simulink model "Wind_Turbine_Model"  (R2023a)
settings: Solver=VariableStepAuto  StartTime=0.0  StopTime=65  RelTol=1e-3
values from neighbouring files (symbols this model uses):
  Cbus = 80e-3*n_wt_agg*u^2    (= 1.33333333333)    [param.m]
  D = 1e-3    (= 0.001)    [param.m]
  f = 50    [param.m]
  Fs = Vs * sqrt(2/3)/(2*pi*f)    [param.m]
  fsw = 4e3    (= 4000)    [param.m]
  Idr_rated = sqrt(2)*Is    [param.m]
  J = 127*n_wt_agg    (= 19050)    [param.m]
  ki_id = (wni^2)*Lr*sigma    (= 3.27733001332)    [param.m]
  ki_idg = (wnig^2)*Lg    (= 0.263189450696)    [param.m]
  ki_iq = ki_id    (= 3.27733001332)    [param.m]
  ki_iqg = ki_idg    (= 0.263189450696)    [param.m]
  ki_v = -300000*n_wt_agg    (= -45000000)    [param.m]
  Kopt = ((0.5*rho*pi*(Radius^5)*Cp_max)/(lambda_opt^3))    (= 296454.198186)    [param.m]
  kp_id = (2*wni*sigma*Lr) - Rr    (= 0.00384733333333)    [param.m]
  kp_idg = ((2*wnig*Lg)-Rg)    (= 0.00167538274858)    [param.m]
  kp_iq = kp_id    (= 0.00384733333333)    [param.m]
  kp_iqg = kp_idg    (= 0.00167538274858)    [param.m]
  kp_v = -1000*n_wt_agg    (= -150000)    [param.m]
  Kpg = 1/(1.5*Vr*sqrt(2/3))    [param.m]
  Kqg = -Kpg    [param.m]
  lambda_opt = 7.2    [param.m]
  Lg = 400e-6 /n_wt_agg    (= 2.66666666667e-06)    [param.m]
  Lm = 2.5e-3 /n_wt_agg    (= 1.66666666667e-05)    [param.m]
  Lr = Lm + Lsi    (= 1.72466666667e-05)    [param.m]
  Ls = Lm + Lsi    (= 1.72466666667e-05)    [param.m]
  Lsi = 0.087e-3 /n_wt_agg    (= 5.8e-07)    [param.m]
  N = 100    [param.m]
  n_wt_agg = 150    [param.m]
  p = 2    [param.m]
  Ps = 2e6*n_wt_agg    (= 300000000)    [param.m]
  Radius = 42    [param.m]
  Rg = 20e-6 /n_wt_agg    (= 1.33333333333e-07)    [param.m]
  rho = 1.225    [param.m]
  Rr = 2.9e-3 /n_wt_agg    (= 1.93333333333e-05)    [param.m]
  Rs = 2.6e-3 /n_wt_agg    (= 1.73333333333e-05)    [param.m]
  sigma = 1 - Lm^2 / (Ls*Lr)    (= 0.0661284179513)    [param.m]
  smax = 1/3    (= 0.333333333333)    [param.m]
  tab_lambda = [0.1:0.01:11.8]    [param.m]
  Ts = 1/fsw/50    (= 5e-06)    [param.m]
  Vbus = 1150/u    (= 3450)    [param.m]
  Vs = 690    [param.m]
undefined symbols (not defined in the file or in its folder): Cp, DiscIntNeverNeededParam
libraries: spsSecondOrderFilterLib x10, simulink x5, spsThreePhaseVIMeasurementLib x4, spsPower3phInstantaneousLib x4, spsPiSectionLineLib x3, spsGroundLib x3, spsThreePhaseTransformerTwoWindingsLib x2, spsThreePhaseProgrammableVoltageSourceLib x2, spsUniversalBridgeLib x2, spsPWMGenerator2LevelLib x2, spsThreePhaseSeriesRLCBranchLib x2, spsAsynchronousMachineSIUnitsLib x1
(part 2 of 2)

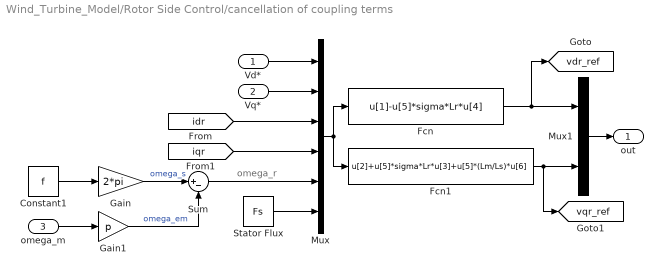
== system Wind_Turbine_Model/Rotor Side Control/cancellation of coupling terms ==
  note: omega_r
  Vd* : Inport
  Vq* : Inport  Port=2
  omega_m : Inport  Port=3
  Constant1 : Constant  Value=f
  Fcn : Fcn  Expr=u[1]-u[5]*sigma*Lr*u[4]
  Fcn1 : Fcn  Expr=u[2]+u[5]*sigma*Lr*u[3]+u[5]*(Lm/Ls)*u[6]
  Gain : Gain  Gain=2*pi
  Gain1 : Gain  Gain=p
  Mux : Mux  Inputs=6
  Mux1 : Mux  Inputs=2
  Stator Flux : Constant  Value=Fs
  Sum : Sum  Inputs=|+-
  out : Outport
  tag scope: vdr_ref=global, vqr_ref=global
  wires:
  Vd*/1 -> Mux/1
  Vq*/1 -> Mux/2
  [idr] -> Mux/3
  [iqr] -> Mux/4
  Sum/1 -> Mux/5
  Stator Flux/1 -> Mux/6
  Constant1/1 -> Gain/1
  Gain/1 -> Sum/1  "omega_s"
  Gain1/1 -> Sum/2  "omega_em"
  omega_m/1 -> Gain1/1
  Mux/1 -> Fcn/1, Fcn1/1
  Mux1/1 -> out/1
  Fcn/1 -> Mux1/1, [vdr_ref]
  Fcn1/1 -> Mux1/2, [vqr_ref]

== system Wind_Turbine_Model/Rotor Side Control/d//q->D//Q ==
  d/q : Inport
  theta : Inport  Port=2
  Fcn : Fcn  Expr=u[1]*cos(u[3])-u[2]*sin(u[3])
  Fcn1 : Fcn  Expr=u[1]*sin(u[3])+u[2]*cos(u[3])
  Mux : Mux  Inputs=2
  Mux1 : Mux  Inputs=2
  D/Q : Outport
  wires:
  Mux/1 -> D/Q/1
  d/q/1 -> Mux1/1
  theta/1 -> Mux1/2
  Fcn/1 -> Mux/1
  Mux1/1 -> Fcn/1, Fcn1/1
  Fcn1/1 -> Mux/2

== system Wind_Turbine_Model/Grid Side Control/angle2/abc->alpha//beta ==
  abc : Inport
  Fcn1 : Fcn  Expr=2/3 * (u[1]-u[2]/2-u[3]/2)
  Fcn2 : Fcn  Expr=2/3 * (u[2] * (sqrt(3)/2) - u[3]*(sqrt(3)/2))
  Mux : Mux  Inputs=2
  alpha/beta : Outport
  wires:
  abc/1 -> Fcn2/1, Fcn1/1
  Mux/1 -> alpha/beta/1
  Fcn1/1 -> Mux/1
  Fcn2/1 -> Mux/2

== system Wind_Turbine_Model/Power Calculations/angle1/abc->alpha//beta ==
  abc : Inport
  Fcn1 : Fcn  Expr=2/3 * (u[1]-u[2]/2-u[3]/2)
  Fcn2 : Fcn  Expr=2/3 * (u[2] * (sqrt(3)/2) - u[3]*(sqrt(3)/2))
  Mux : Mux  Inputs=2
  alpha/beta : Outport
  wires:
  Fcn2/1 -> Mux/2
  Fcn1/1 -> Mux/1
  Mux/1 -> alpha/beta/1
  abc/1 -> Fcn1/1, Fcn2/1

== system Wind_Turbine_Model/Power Calculations/angle2/abc->alpha//beta ==
  abc : Inport
  Fcn1 : Fcn  Expr=2/3 * (u[1]-u[2]/2-u[3]/2)
  Fcn2 : Fcn  Expr=2/3 * (u[2] * (sqrt(3)/2) - u[3]*(sqrt(3)/2))
  Mux : Mux  Inputs=2
  alpha/beta : Outport
  wires:
  abc/1 -> Fcn2/1, Fcn1/1
  Mux/1 -> alpha/beta/1
  Fcn1/1 -> Mux/1
  Fcn2/1 -> Mux/2

== system Wind_Turbine_Model/Rotor Side Control/angle/abc->alpha//beta ==
  abc : Inport
  Fcn1 : Fcn  Expr=2/3 * (u[1]-u[2]/2-u[3]/2)
  Fcn2 : Fcn  Expr=2/3 * (u[2] * (sqrt(3)/2) - u[3]*(sqrt(3)/2))
  Mux : Mux  Inputs=2
  alpha/beta : Outport
  wires:
  abc/1 -> Fcn2/1, Fcn1/1
  Mux/1 -> alpha/beta/1
  Fcn1/1 -> Mux/1
  Fcn2/1 -> Mux/2
